simulink model "GreenCraneSimulator"  (R2021b)
settings: Solver=ode23  StartTime=0.0  StopTime=25  FixedStep=0.0001  RelTol=1e-3
undefined symbols (not defined in the file): Annulus_area, beta_F, Bore_area, cyl_c_end, cyl_c_visc, cyl_CH_stat, cyl_F_coul, cyl_FH_stat, cyl_gamma, cyl_k_end, DiscIntNeverNeededParam, dr_dcv, Eff_Bulk_On, eta_air, k_cv, k_DCV_PA, k_DCV_PB, k_DCV_T, k_ocv, K_oil, k_tanh, kappa_air, mu_ocv, OL_pa, OL_pb, p0_A, p0_A1, p0_B, p_cv_fo, p_cv_set, p_ocv_fo, p_ocv_set, p_pc_set, p_R, p_S, patm, Stroke, tau_ocv, tau_pc, tCycle, UL_at, UL_bt, V_CH_A, V_CH_A1, V_CH_B, v_cyl_0, wn_dcv, X, x_cyl_0, Y, Z
libraries: sm_lib x25, nesl_utility x4, simulink x1
(part 1 of 2)
settings Model: Creator=hagen  LastModifiedBy=danielh

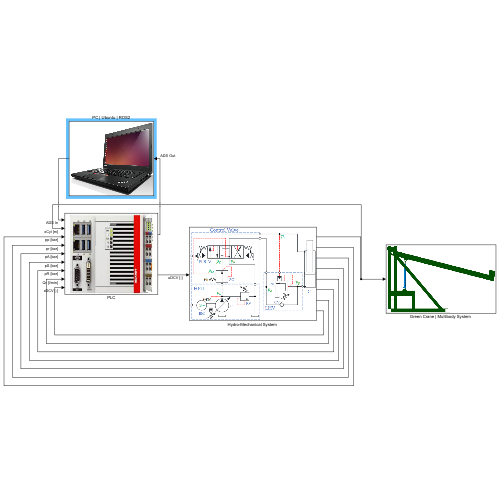
[thumbnail: Simulink's stored preview of the top-level diagram]
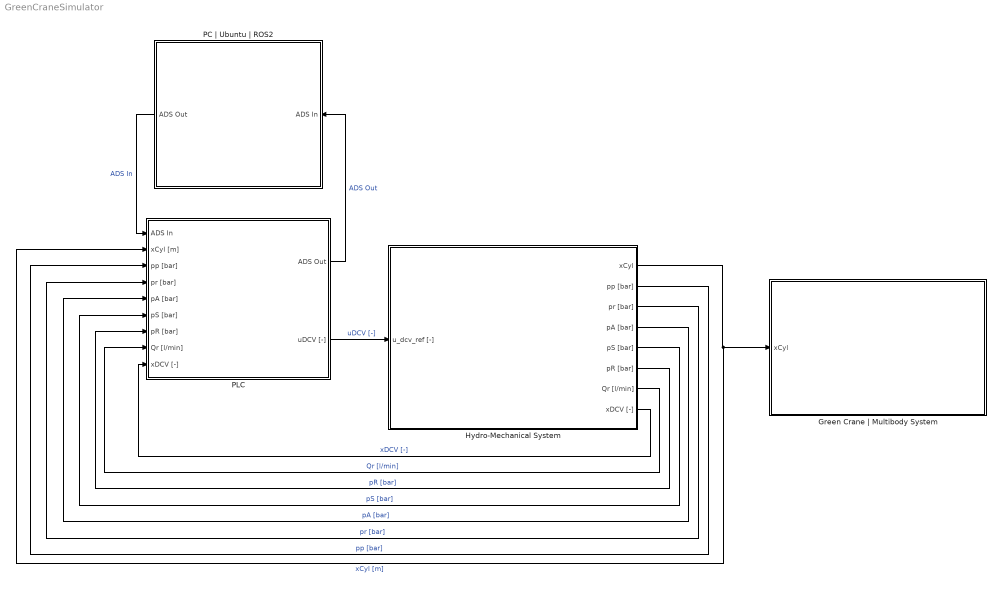
== system GreenCraneSimulator ==
  "Green Crane | Multibody System " : Subsystem
      mask Display: image('..\Simulink Model MAS418 LAB #11\Figures\GreenCrane.png'); % Use "Edit Image" on toolstrip to change.
  "Hydro-Mechanical System " : Subsystem
      mask Display: image('..\Simulink Model MAS418 LAB #11\Figures\HydroMechanicalSystem.png'); % Use "Edit Image" on toolstrip to change.
  PC | Ubuntu | ROS2 : Subsystem
      mask Display: image('..\Simulink Model MAS418 LAB #11\Figures\PC.png'); % Use "Edit Image" on toolstrip to change.
  PLC : Subsystem
      mask Display: image('..\Simulink Model MAS418 LAB #11\Figures\PLC.jpg'); % Use "Edit Image" on toolstrip to change.
  wires:
  PC | Ubuntu | ROS2/1(ADS Out) -> PLC/1(ADS In)  "ADS In"
  "Hydro-Mechanical System "/2(pp [bar]) -> PLC/3(pp [bar])  "pp [bar]"
  "Hydro-Mechanical System "/3(pr [bar]) -> PLC/4(pr [bar])  "pr [bar]"
  PLC/1(ADS Out) -> PC | Ubuntu | ROS2/1(ADS In)  "ADS Out"
  PLC/2(uDCV [-]) -> "Hydro-Mechanical System "/1(u_dcv_ref [-])  "uDCV [-]"
  "Hydro-Mechanical System "/4(pA [bar]) -> PLC/5(pA [bar])  "pA [bar]"
  "Hydro-Mechanical System "/8(xDCV [-]) -> PLC/9(xDCV [-])  "xDCV [-]"
  "Hydro-Mechanical System "/7(Qr [l/min]) -> PLC/8(Qr [l/min])  "Qr [l/min]"
  "Hydro-Mechanical System "/6(pR [bar]) -> PLC/7(pR [bar])  "pR [bar]"
  "Hydro-Mechanical System "/5(pS [bar]) -> PLC/6(pS [bar])  "pS [bar]"
  "Hydro-Mechanical System "/1(xCyl) -> PLC/2(xCyl [m]), "Green Crane | Multibody System "/1(xCyl)  "xCyl [m]"

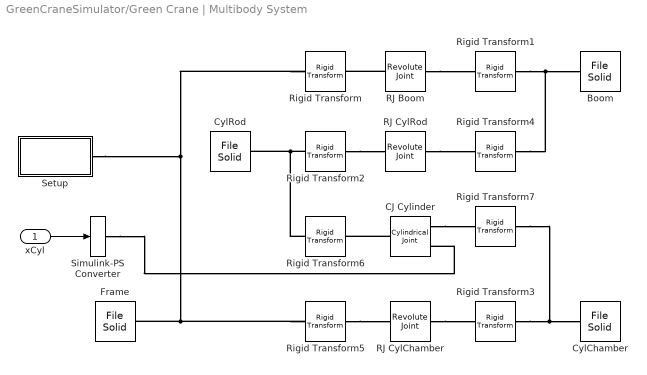
== system GreenCraneSimulator/Green Crane | Multibody System  ==
  xCyl : Inport
  Boom : sm_lib/Body Elements/File Solid  ExtGeomFileName=..\Simulink Model MAS418 LAB #7\CAD\Boom.STL  UnitType=Custom  ExtGeomFileUnits=mm  StepReaderType=HEX  ExportConvexHullGeometry=off  InertiaType=CalculateFromGeometry  Mass=1  MassUnits=kg  CenterOfMass=[0 0 0]  CenterOfMassUnits=m  MomentsOfInertia=[1 1 1]  MomentsOfInertiaUnits=kg*m^2  ProductsOfInertia=[0 0 0]  ProductsOfInertiaUnits=kg*m^2  BasedOnType=Density  Density=1000  DensityUnits=kg/m^3  DoExposeReferenceFrame=off  SerializedFrames=<Frames><Frame><Id>Frame1</Id><Value><Name>F1</Name><Origin><Source>CenterOfMassFrame</Source><FeatureName></FeatureName></Origin><PrimaryAxis><DefinedDirection>+Y</DefinedDirection><Source>ReferenceFrame</Source><SourceDirection>-Z</SourceDirection><FeatureName></FeatureName></PrimaryAxis><SecondaryAxis><DefinedDirection>+X</DefinedDirection><Source>ReferenceFrame</Source><SourceDirection>+X</SourceDirection><FeatureName></FeatureName></SecondaryAxis></Value></Frame></Frames>  GraphicType=FromGeometry  MarkerShape=Sphere  MarkerSize=10  GraphicVisPropType=SimpleVisualProperties  GraphicDiffuseColor=[0.0 0.4 0.0]  GraphicSpecularColor=[0.5 0.5 0.5 1.0]  GraphicAmbientColor=[0.15 0.15 0.15 1.0]  GraphicEmissiveColor=[0.0 0.0 0.0 1.0]  GraphicShininess=75  GraphicOpacity=1.0
  CJ Cylinder : sm_lib/Joints/Cylindrical Joint  JointMode=Normal  SenseConstraintForce=off  SenseConstraintForceX=off  SenseConstraintForceY=off  SenseConstraintForceZ=off  SenseConstraintTorque=off  SenseConstraintTorqueX=off  SenseConstraintTorqueY=off  SenseConstraintTorqueZ=off  SenseTotalForce=off  SenseTotalForceX=off  SenseTotalForceY=off  SenseTotalForceZ=off  SenseTotalTorque=off  SenseTotalTorqueX=off  SenseTotalTorqueY=off  SenseTotalTorqueZ=off  CompositeWrenchDir=FollowerOnBase  CompositeWrenchFrame=BaseFrame  PzEquilibriumPosition=0  PzEquilibriumPositionUnits=m  PzSpringStiffness=0  PzSpringStiffnessUnits=N/m  PzDampingCoefficient=0  PzDampingCoefficientUnits=N/(m/s)  PzTorqueActuationMode=ComputedTorque  PzMotionActuationMode=InputMotion  PzSensePosition=off  PzSenseVelocity=off  PzSenseAcceleration=off  PzSenseTorqueForce=off  PzSenseLowerLimitTorqueForce=off  PzSenseUpperLimitTorqueForce=off  PzLowerLimitSpecify=off  PzLowerLimitBound=-1  PzLowerLimitBoundUnits=m  PzLowerLimitStiffness=1e6  PzLowerLimitStiffnessUnits=N/m  PzLowerLimitDamping=1e3  PzLowerLimitDampingUnits=N/(m/s)  PzLowerLimitTransitionRegionWidth=1e-4  PzLowerLimitTransitionRegionWidthUnits=m  PzUpperLimitSpecify=off  PzUpperLimitBound=1  PzUpperLimitBoundUnits=m  PzUpperLimitStiffness=1e6  PzUpperLimitStiffnessUnits=N/m  PzUpperLimitDamping=1e3  PzUpperLimitDampingUnits=N/(m/s)  PzUpperLimitTransitionRegionWidth=1e-4  PzUpperLimitTransitionRegionWidthUnits=m  PzPositionTargetSpecify=on  PzPositionTargetPriority=High  PzPositionTargetValue=x_cyl_0  PzPositionTargetValueUnits=m  PzVelocityTargetSpecify=off  PzVelocityTargetPriority=High  PzVelocityTargetValue=0  PzVelocityTargetValueUnits=m/s  RzEquilibriumPosition=0  RzEquilibriumPositionUnits=deg  RzSpringStiffness=0  RzSpringStiffnessUnits=N*m/deg  RzDampingCoefficient=0  RzDampingCoefficientUnits=N*m/(deg/s)  RzTorqueActuationMode=NoTorque  RzMotionActuationMode=ComputedMotion  RzSensePosition=off  RzSenseVelocity=off  RzSenseAcceleration=off  RzSenseTorqueForce=off  RzSenseLowerLimitTorqueForce=off  RzSenseUpperLimitTorqueForce=off  RzLowerLimitSpecify=off  RzLowerLimitBound=-90  RzLowerLimitBoundUnits=deg  RzLowerLimitStiffness=1e4  RzLowerLimitStiffnessUnits=N*m/deg  RzLowerLimitDamping=10  RzLowerLimitDampingUnits=N*m/(deg/s)  RzLowerLimitTransitionRegionWidth=0.1  RzLowerLimitTransitionRegionWidthUnits=deg  RzUpperLimitSpecify=off  RzUpperLimitBound=90  RzUpperLimitBoundUnits=deg  RzUpperLimitStiffness=1e4  RzUpperLimitStiffnessUnits=N*m/deg  RzUpperLimitDamping=10  RzUpperLimitDampingUnits=N*m/(deg/s)  RzUpperLimitTransitionRegionWidth=0.1  RzUpperLimitTransitionRegionWidthUnits=deg  RzPositionTargetSpecify=off  RzPositionTargetPriority=High  RzPositionTargetValue=0  RzPositionTargetValueUnits=deg  RzVelocityTargetSpecify=off  RzVelocityTargetPriority=High  RzVelocityTargetValue=0  RzVelocityTargetValueUnits=deg/s
  CylChamber : sm_lib/Body Elements/File Solid  ExtGeomFileName=..\Simulink Model MAS418 LAB #7\CAD\cyl_chamber.STL  UnitType=Custom  ExtGeomFileUnits=mm  StepReaderType=HEX  ExportConvexHullGeometry=off  InertiaType=CalculateFromGeometry  Mass=1  MassUnits=kg  CenterOfMass=[0 0 0]  CenterOfMassUnits=m  MomentsOfInertia=[1 1 1]  MomentsOfInertiaUnits=kg*m^2  ProductsOfInertia=[0 0 0]  ProductsOfInertiaUnits=kg*m^2  BasedOnType=Density  Density=1000  DensityUnits=kg/m^3  DoExposeReferenceFrame=off  SerializedFrames=<Frames><Frame><Id>Frame1</Id><Value><Name>F1</Name><Origin><Source>CenterOfMassFrame</Source><FeatureName></FeatureName></Origin><PrimaryAxis><DefinedDirection>+Y</DefinedDirection><Source>ReferenceFrame</Source><SourceDirection>-Z</SourceDirection><FeatureName></FeatureName></PrimaryAxis><SecondaryAxis><DefinedDirection>+X</DefinedDirection><Source>ReferenceFrame</Source><SourceDirection>+X</SourceDirection><FeatureName></FeatureName></SecondaryAxis></Value></Frame></Frames>  GraphicType=FromGeometry  MarkerShape=Sphere  MarkerSize=10  GraphicVisPropType=SimpleVisualProperties  GraphicDiffuseColor=[0.0 0.6 1.0]  GraphicSpecularColor=[0.5 0.5 0.5 1.0]  GraphicAmbientColor=[0.15 0.15 0.15 1.0]  GraphicEmissiveColor=[0.0 0.0 0.0 1.0]  GraphicShininess=75  GraphicOpacity=1.0
  CylRod : sm_lib/Body Elements/File Solid  ExtGeomFileName=..\Simulink Model MAS418 LAB #7\CAD\cyl_rod.STL  UnitType=Custom  ExtGeomFileUnits=mm  StepReaderType=HEX  ExportConvexHullGeometry=off  InertiaType=CalculateFromGeometry  Mass=1  MassUnits=kg  CenterOfMass=[0 0 0]  CenterOfMassUnits=m  MomentsOfInertia=[1 1 1]  MomentsOfInertiaUnits=kg*m^2  ProductsOfInertia=[0 0 0]  ProductsOfInertiaUnits=kg*m^2  BasedOnType=Density  Density=1000  DensityUnits=kg/m^3  DoExposeReferenceFrame=off  SerializedFrames=<Frames><Frame><Id>Frame1</Id><Value><Name>F1</Name><Origin><Source>CenterOfMassFrame</Source><FeatureName></FeatureName></Origin><PrimaryAxis><DefinedDirection>+Y</DefinedDirection><Source>ReferenceFrame</Source><SourceDirection>-Z</SourceDirection><FeatureName></FeatureName></PrimaryAxis><SecondaryAxis><DefinedDirection>+X</DefinedDirection><Source>ReferenceFrame</Source><SourceDirection>+X</SourceDirection><FeatureName></FeatureName></SecondaryAxis></Value></Frame></Frames>  GraphicType=FromGeometry  MarkerShape=Sphere  MarkerSize=10  GraphicVisPropType=SimpleVisualProperties  GraphicDiffuseColor=[0.8 0.8 0.8]  GraphicSpecularColor=[0.5 0.5 0.5 1.0]  GraphicAmbientColor=[0.15 0.15 0.15 1.0]  GraphicEmissiveColor=[0.0 0.0 0.0 1.0]  GraphicShininess=75  GraphicOpacity=1.0
  Frame : sm_lib/Body Elements/File Solid  ExtGeomFileName=..\Simulink Model MAS418 LAB #7\CAD\Frame.STL  UnitType=Custom  ExtGeomFileUnits=mm  StepReaderType=HEX  ExportConvexHullGeometry=off  InertiaType=CalculateFromGeometry  Mass=1  MassUnits=kg  CenterOfMass=[0 0 0]  CenterOfMassUnits=m  MomentsOfInertia=[1 1 1]  MomentsOfInertiaUnits=kg*m^2  ProductsOfInertia=[0 0 0]  ProductsOfInertiaUnits=kg*m^2  BasedOnType=Density  Density=1000  DensityUnits=kg/m^3  DoExposeReferenceFrame=off  SerializedFrames=<Frames><Frame><Id>Frame1</Id><Value><Name>F1</Name><Origin><Source>CenterOfMassFrame</Source><FeatureName></FeatureName></Origin><PrimaryAxis><DefinedDirection>-Y</DefinedDirection><Source>ReferenceFrame</Source><SourceDirection>+Z</SourceDirection><FeatureName></FeatureName></PrimaryAxis><SecondaryAxis><DefinedDirection>+X</DefinedDirection><Source>ReferenceFrame</Source><SourceDirection>+X</SourceDirection><FeatureName></FeatureName></SecondaryAxis></Value></Frame></Frames>  GraphicType=FromGeometry  MarkerShape=Sphere  MarkerSize=10  GraphicVisPropType=SimpleVisualProperties  GraphicDiffuseColor=[0.0 0.4 0.0]  GraphicSpecularColor=[0.5 0.5 0.5 1.0]  GraphicAmbientColor=[0.15 0.15 0.15 1.0]  GraphicEmissiveColor=[0.0 0.0 0.0 1.0]  GraphicShininess=75  GraphicOpacity=1.0
  RJ Boom : sm_lib/Joints/Revolute Joint  JointMode=Normal  SenseConstraintForce=off  SenseConstraintForceX=off  SenseConstraintForceY=off  SenseConstraintForceZ=off  SenseConstraintTorque=off  SenseConstraintTorqueX=off  SenseConstraintTorqueY=off  SenseConstraintTorqueZ=off  SenseTotalForce=off  SenseTotalForceX=off  SenseTotalForceY=off  SenseTotalForceZ=off  SenseTotalTorque=off  SenseTotalTorqueX=off  SenseTotalTorqueY=off  SenseTotalTorqueZ=off  CompositeWrenchDir=FollowerOnBase  CompositeWrenchFrame=BaseFrame  EquilibriumPosition=0  EquilibriumPositionUnits=deg  SpringStiffness=0  SpringStiffnessUnits=N*m/deg  DampingCoefficient=0  DampingCoefficientUnits=N*m/(deg/s)  TorqueActuationMode=NoTorque  MotionActuationMode=ComputedMotion  SensePosition=off  SenseVelocity=off  SenseAcceleration=off  SenseTorqueForce=off  SenseLowerLimitTorqueForce=off  SenseUpperLimitTorqueForce=off  LowerLimitSpecify=off  LowerLimitBound=-90  LowerLimitBoundUnits=deg  LowerLimitStiffness=1e4  LowerLimitStiffnessUnits=N*m/deg  LowerLimitDamping=10  LowerLimitDampingUnits=N*m/(deg/s)  LowerLimitTransitionRegionWidth=0.1  LowerLimitTransitionRegionWidthUnits=deg  UpperLimitSpecify=off  UpperLimitBound=90  UpperLimitBoundUnits=deg  UpperLimitStiffness=1e4  UpperLimitStiffnessUnits=N*m/deg  UpperLimitDamping=10  UpperLimitDampingUnits=N*m/(deg/s)  UpperLimitTransitionRegionWidth=0.1  UpperLimitTransitionRegionWidthUnits=deg  PositionTargetSpecify=off  PositionTargetPriority=High  PositionTargetValue=0  PositionTargetValueUnits=deg  VelocityTargetSpecify=off  VelocityTargetPriority=High  VelocityTargetValue=0  VelocityTargetValueUnits=deg/s
  RJ CylChamber : sm_lib/Joints/Revolute Joint  JointMode=Normal  SenseConstraintForce=off  SenseConstraintForceX=off  SenseConstraintForceY=off  SenseConstraintForceZ=off  SenseConstraintTorque=off  SenseConstraintTorqueX=off  SenseConstraintTorqueY=off  SenseConstraintTorqueZ=off  SenseTotalForce=off  SenseTotalForceX=off  SenseTotalForceY=off  SenseTotalForceZ=off  SenseTotalTorque=off  SenseTotalTorqueX=off  SenseTotalTorqueY=off  SenseTotalTorqueZ=off  CompositeWrenchDir=FollowerOnBase  CompositeWrenchFrame=BaseFrame  EquilibriumPosition=0  EquilibriumPositionUnits=deg  SpringStiffness=0  SpringStiffnessUnits=N*m/deg  DampingCoefficient=0  DampingCoefficientUnits=N*m/(deg/s)  TorqueActuationMode=NoTorque  MotionActuationMode=ComputedMotion  SensePosition=off  SenseVelocity=off  SenseAcceleration=off  SenseTorqueForce=off  SenseLowerLimitTorqueForce=off  SenseUpperLimitTorqueForce=off  LowerLimitSpecify=off  LowerLimitBound=-90  LowerLimitBoundUnits=deg  LowerLimitStiffness=1e4  LowerLimitStiffnessUnits=N*m/deg  LowerLimitDamping=10  LowerLimitDampingUnits=N*m/(deg/s)  LowerLimitTransitionRegionWidth=0.1  LowerLimitTransitionRegionWidthUnits=deg  UpperLimitSpecify=off  UpperLimitBound=90  UpperLimitBoundUnits=deg  UpperLimitStiffness=1e4  UpperLimitStiffnessUnits=N*m/deg  UpperLimitDamping=10  UpperLimitDampingUnits=N*m/(deg/s)  UpperLimitTransitionRegionWidth=0.1  UpperLimitTransitionRegionWidthUnits=deg  PositionTargetSpecify=off  PositionTargetPriority=High  PositionTargetValue=0  PositionTargetValueUnits=deg  VelocityTargetSpecify=off  VelocityTargetPriority=High  VelocityTargetValue=0  VelocityTargetValueUnits=deg/s
  RJ CylRod : sm_lib/Joints/Revolute Joint  JointMode=Normal  SenseConstraintForce=off  SenseConstraintForceX=off  SenseConstraintForceY=off  SenseConstraintForceZ=off  SenseConstraintTorque=off  SenseConstraintTorqueX=off  SenseConstraintTorqueY=off  SenseConstraintTorqueZ=off  SenseTotalForce=off  SenseTotalForceX=off  SenseTotalForceY=off  SenseTotalForceZ=off  SenseTotalTorque=off  SenseTotalTorqueX=off  SenseTotalTorqueY=off  SenseTotalTorqueZ=off  CompositeWrenchDir=FollowerOnBase  CompositeWrenchFrame=BaseFrame  EquilibriumPosition=0  EquilibriumPositionUnits=deg  SpringStiffness=0  SpringStiffnessUnits=N*m/deg  DampingCoefficient=0  DampingCoefficientUnits=N*m/(deg/s)  TorqueActuationMode=NoTorque  MotionActuationMode=ComputedMotion  SensePosition=off  SenseVelocity=off  SenseAcceleration=off  SenseTorqueForce=off  SenseLowerLimitTorqueForce=off  SenseUpperLimitTorqueForce=off  LowerLimitSpecify=off  LowerLimitBound=-90  LowerLimitBoundUnits=deg  LowerLimitStiffness=1e4  LowerLimitStiffnessUnits=N*m/deg  LowerLimitDamping=10  LowerLimitDampingUnits=N*m/(deg/s)  LowerLimitTransitionRegionWidth=0.1  LowerLimitTransitionRegionWidthUnits=deg  UpperLimitSpecify=off  UpperLimitBound=90  UpperLimitBoundUnits=deg  UpperLimitStiffness=1e4  UpperLimitStiffnessUnits=N*m/deg  UpperLimitDamping=10  UpperLimitDampingUnits=N*m/(deg/s)  UpperLimitTransitionRegionWidth=0.1  UpperLimitTransitionRegionWidthUnits=deg  PositionTargetSpecify=off  PositionTargetPriority=High  PositionTargetValue=0  PositionTargetValueUnits=deg  VelocityTargetSpecify=off  VelocityTargetPriority=High  VelocityTargetValue=0  VelocityTargetValueUnits=deg/s
  Rigid Transform : sm_lib/Frames and Transforms/Rigid Transform  TranslationMethod=Cartesian  TranslationStandardOffset=0  TranslationLengthUnit=mm  TranslationStandardAxis=+Z  TranslationCartesianOffset=[-568.76 0 1179.93]  TranslationROffset=0  TranslationROffsetUnits=m  TranslationZOffset=0  TranslationZOffsetUnits=m  TranslationThetaOffset=0  TranslationThetaOffsetUnits=deg  RotationMethod=StandardAxis  RotationAngleUnits=deg  RotationStandardAxis=+X  RotationAngle=90  RotationArbitraryAxis=[0 0 1]  FollAlignAxisA=+X  BaseAlignAxisA=+Y  FollAlignAxisB=+Y  BaseAlignAxisB=+Z  RotationSequenceAxes=FollowerAxes  RotationSequence=XYX  RotationSequenceAngles=[0 0 0]  RotationSequenceAnglesUnits=deg  RotationMatrix=[1 0 0; 0 1 0; 0 0 1]
  Rigid Transform1 : sm_lib/Frames and Transforms/Rigid Transform  TranslationMethod=Cartesian  TranslationStandardOffset=0  TranslationLengthUnit=mm  TranslationStandardAxis=+Z  TranslationCartesianOffset=[-3108.36 0 -63.43]  TranslationROffset=0  TranslationROffsetUnits=m  TranslationZOffset=0  TranslationZOffsetUnits=m  TranslationThetaOffset=0  TranslationThetaOffsetUnits=deg  RotationMethod=StandardAxis  RotationAngleUnits=deg  RotationStandardAxis=+X  RotationAngle=90  RotationArbitraryAxis=[0 0 1]  FollAlignAxisA=+X  BaseAlignAxisA=+Y  FollAlignAxisB=+Y  BaseAlignAxisB=+Z  RotationSequenceAxes=FollowerAxes  RotationSequence=XYX  RotationSequenceAngles=[0 0 0]  RotationSequenceAnglesUnits=deg  RotationMatrix=[1 0 0; 0 1 0; 0 0 1]
  Rigid Transform2 : sm_lib/Frames and Transforms/Rigid Transform  TranslationMethod=Cartesian  TranslationStandardOffset=0  TranslationLengthUnit=mm  TranslationStandardAxis=+Z  TranslationCartesianOffset=[0 0 292.43]  TranslationROffset=0  TranslationROffsetUnits=m  TranslationZOffset=0  TranslationZOffsetUnits=m  TranslationThetaOffset=0  TranslationThetaOffsetUnits=deg  RotationMethod=StandardAxis  RotationAngleUnits=deg  RotationStandardAxis=+X  RotationAngle=90  RotationArbitraryAxis=[0 0 1]  FollAlignAxisA=+X  BaseAlignAxisA=+Y  FollAlignAxisB=+Y  BaseAlignAxisB=+Z  RotationSequenceAxes=FollowerAxes  RotationSequence=XYX  RotationSequenceAngles=[0 0 0]  RotationSequenceAnglesUnits=deg  RotationMatrix=[1 0 0; 0 1 0; 0 0 1]
  Rigid Transform3 : sm_lib/Frames and Transforms/Rigid Transform  TranslationMethod=Cartesian  TranslationStandardOffset=0  TranslationLengthUnit=mm  TranslationStandardAxis=+Z  TranslationCartesianOffset=[0 0 -260.99]  TranslationROffset=0  TranslationROffsetUnits=m  TranslationZOffset=0  TranslationZOffsetUnits=m  TranslationThetaOffset=0  TranslationThetaOffsetUnits=deg  RotationMethod=StandardAxis  RotationAngleUnits=deg  RotationStandardAxis=+X  RotationAngle=90  RotationArbitraryAxis=[0 0 1]  FollAlignAxisA=+X  BaseAlignAxisA=+Y  FollAlignAxisB=+Y  BaseAlignAxisB=+Z  RotationSequenceAxes=FollowerAxes  RotationSequence=XYX  RotationSequenceAngles=[0 0 0]  RotationSequenceAnglesUnits=deg  RotationMatrix=[1 0 0; 0 1 0; 0 0 1]
  Rigid Transform4 : sm_lib/Frames and Transforms/Rigid Transform  TranslationMethod=Cartesian  TranslationStandardOffset=0  TranslationLengthUnit=mm  TranslationStandardAxis=+Z  TranslationCartesianOffset=[-2613.52 0 -196.43]  TranslationROffset=0  TranslationROffsetUnits=m  TranslationZOffset=0  TranslationZOffsetUnits=m  TranslationThetaOffset=0  TranslationThetaOffsetUnits=deg  RotationMethod=StandardAxis  RotationAngleUnits=deg  RotationStandardAxis=+X  RotationAngle=90  RotationArbitraryAxis=[0 0 1]  FollAlignAxisA=+X  BaseAlignAxisA=+Y  FollAlignAxisB=+Y  BaseAlignAxisB=+Z  RotationSequenceAxes=FollowerAxes  RotationSequence=XYX  RotationSequenceAngles=[0 0 0]  RotationSequenceAnglesUnits=deg  RotationMatrix=[1 0 0; 0 1 0; 0 0 1]
  Rigid Transform5 : sm_lib/Frames and Transforms/Rigid Transform  TranslationMethod=Cartesian  TranslationStandardOffset=0  TranslationLengthUnit=mm  TranslationStandardAxis=+Z  TranslationCartesianOffset=[-141.76 0 122.93]  TranslationROffset=0  TranslationROffsetUnits=m  TranslationZOffset=0  TranslationZOffsetUnits=m  TranslationThetaOffset=0  TranslationThetaOffsetUnits=deg  RotationMethod=StandardAxis  RotationAngleUnits=deg  RotationStandardAxis=+X  RotationAngle=90  RotationArbitraryAxis=[0 0 1]  FollAlignAxisA=+X  BaseAlignAxisA=+Y  FollAlignAxisB=+Y  BaseAlignAxisB=+Z  RotationSequenceAxes=FollowerAxes  RotationSequence=XYX  RotationSequenceAngles=[0 0 0]  RotationSequenceAnglesUnits=deg  RotationMatrix=[1 0 0; 0 1 0; 0 0 1]
  Rigid Transform6 : sm_lib/Frames and Transforms/Rigid Transform  TranslationMethod=Cartesian  TranslationStandardOffset=0  TranslationLengthUnit=mm  TranslationStandardAxis=+Z  TranslationCartesianOffset=[0 0 -307.79]  TranslationROffset=0  TranslationROffsetUnits=m  TranslationZOffset=0  TranslationZOffsetUnits=m  TranslationThetaOffset=0  TranslationThetaOffsetUnits=deg  RotationMethod=None  RotationAngleUnits=deg  RotationStandardAxis=-X  RotationAngle=90  RotationArbitraryAxis=[0 0 1]  FollAlignAxisA=+X  BaseAlignAxisA=+Y  FollAlignAxisB=+Y  BaseAlignAxisB=+Z  RotationSequenceAxes=FollowerAxes  RotationSequence=XYX  RotationSequenceAngles=[0 0 0]  RotationSequenceAnglesUnits=deg  RotationMatrix=[1 0 0; 0 1 0; 0 0 1]
  Rigid Transform7 : sm_lib/Frames and Transforms/Rigid Transform  TranslationMethod=Cartesian  TranslationStandardOffset=0  TranslationLengthUnit=mm  TranslationStandardAxis=+Z  TranslationCartesianOffset=[0 0 -88.99]  TranslationROffset=0  TranslationROffsetUnits=m  TranslationZOffset=0  TranslationZOffsetUnits=m  TranslationThetaOffset=0  TranslationThetaOffsetUnits=deg  RotationMethod=None  RotationAngleUnits=deg  RotationStandardAxis=-X  RotationAngle=90  RotationArbitraryAxis=[0 0 1]  FollAlignAxisA=+X  BaseAlignAxisA=+Y  FollAlignAxisB=+Y  BaseAlignAxisB=+Z  RotationSequenceAxes=FollowerAxes  RotationSequence=XYX  RotationSequenceAngles=[0 0 0]  RotationSequenceAnglesUnits=deg  RotationMatrix=[1 0 0; 0 1 0; 0 0 1]
  Setup : Subsystem
  Simulink-PS Converter : nesl_utility/Simulink-PS Converter  PhysicalDomain=network_engine_domain  SubClassName=ps_input  LeftPortType=input  RightPortType=output  PseudoPeriodic=off  Frequencies=[]  NoiseDistribution=none  NoiseParameters=[]  Unit=1  AffineConversion=off  FilteringAndDerivatives=filter  SimscapeFilterOrder=2  InputFilterTimeConstant=0.001  UdotUserProvided=0
      settings: SourceProductBaseCode=PW,SS
  wires:
  xCyl/1 -> Simulink-PS Converter/1
  connections:
  Rigid Transform/LConn1 -- Rigid Transform5/LConn1 -- Frame/LConn1 -- Setup/RConn1
  CJ Cylinder/LConn1 -- Rigid Transform7/RConn1
  Rigid Transform2/LConn1 -- Rigid Transform6/LConn1 -- CylRod/LConn1
  Rigid Transform1/LConn1 -- Rigid Transform4/LConn1 -- Boom/LConn1
  Rigid Transform3/LConn1 -- Rigid Transform7/LConn1 -- CylChamber/LConn1
  RJ CylChamber/RConn1 -- Rigid Transform3/RConn1
  RJ Boom/LConn1 -- Rigid Transform/RConn1
  CJ Cylinder/RConn1 -- Rigid Transform6/RConn1
  RJ Boom/RConn1 -- Rigid Transform1/RConn1
  Simulink-PS Converter/RConn1 -- CJ Cylinder/LConn2
  Rigid Transform5/RConn1 -- RJ CylChamber/LConn1
  RJ CylRod/LConn1 -- Rigid Transform4/RConn1
  Rigid Transform2/RConn1 -- RJ CylRod/RConn1

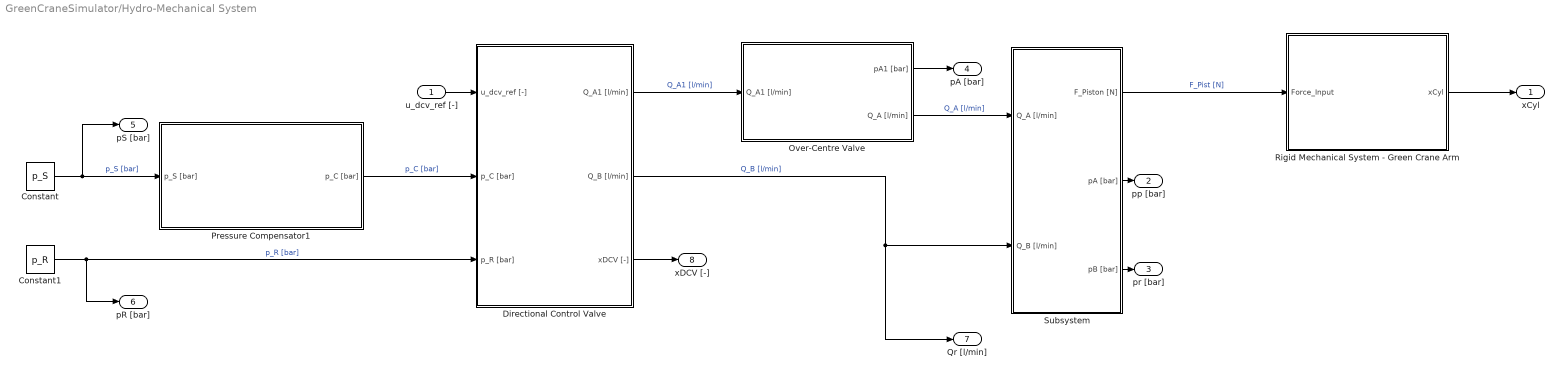
== system GreenCraneSimulator/Hydro-Mechanical System  ==
  u_dcv_ref [-] : Inport
  Constant : Constant  Value=p_S
  Constant1 : Constant  Value=p_R
  Directional Control Valve : Subsystem
      mask Display: disp('{\bf\fontsize{22}Directional\newline Control Valve}', 'texmode','on');
  Over-Centre Valve : Subsystem
      mask Display: disp('{\bf\fontsize{22}Load-Holding\newline Valve}', 'texmode','on');
  Pressure Compensator1 : Subsystem
      mask Display: disp('{\bf\fontsize{22}Pressure\newline Compensator}', 'texmode','on');
  Rigid Mechanical System - Green Crane Arm : Subsystem  VariantControl=Rigid_model
  Subsystem : Subsystem
      mask Display: disp('{\bf\fontsize{22} Hydraulic \newline Cylinder}', 'texmode','on');
  xCyl : Outport
  pp [bar] : Outport  Port=2  VectorParamsAs1DForOutWhenUnconnected=off
  pr [bar] : Outport  Port=3  VectorParamsAs1DForOutWhenUnconnected=off
  pA [bar] : Outport  Port=4  VectorParamsAs1DForOutWhenUnconnected=off
  pS [bar] : Outport  Port=5  VectorParamsAs1DForOutWhenUnconnected=off
  pR [bar] : Outport  Port=6  VectorParamsAs1DForOutWhenUnconnected=off
  Qr [l/min] : Outport  Port=7  VectorParamsAs1DForOutWhenUnconnected=off
  xDCV [-] : Outport  Port=8  VectorParamsAs1DForOutWhenUnconnected=off
  wires:
  Subsystem/1(F_Piston [N]) -> Rigid Mechanical System - Green Crane Arm/1(Force_Input)  "F_Pist [N]"
  Constant/1 -> pS [bar]/1, Pressure Compensator1/1(p_S [bar])  "p_S [bar]"
  Pressure Compensator1/1(p_C [bar]) -> Directional Control Valve/2(p_C [bar])  "p_C [bar]"
  Directional Control Valve/2(Q_B [l/min]) -> Qr [l/min]/1, Subsystem/2(Q_B [l/min])  "Q_B [l/min]"
  u_dcv_ref [-]/1 -> Directional Control Valve/1(u_dcv_ref [-])
  Over-Centre Valve/2(Q_A [l/min]) -> Subsystem/1(Q_A [l/min])  "Q_A [l/min]"
  Constant1/1 -> pR [bar]/1, Directional Control Valve/3(p_R [bar])  "p_R [bar]"
  Directional Control Valve/1(Q_A1 [l/min]) -> Over-Centre Valve/1(Q_A1 [l/min])  "Q_A1 [l/min]"
  Rigid Mechanical System - Green Crane Arm/1(xCyl) -> xCyl/1
  Subsystem/2(pA [bar]) -> pp [bar]/1
  Subsystem/3(pB [bar]) -> pr [bar]/1
  Over-Centre Valve/1(pA1 [bar]) -> pA [bar]/1
  Directional Control Valve/3(xDCV [-]) -> xDCV [-]/1

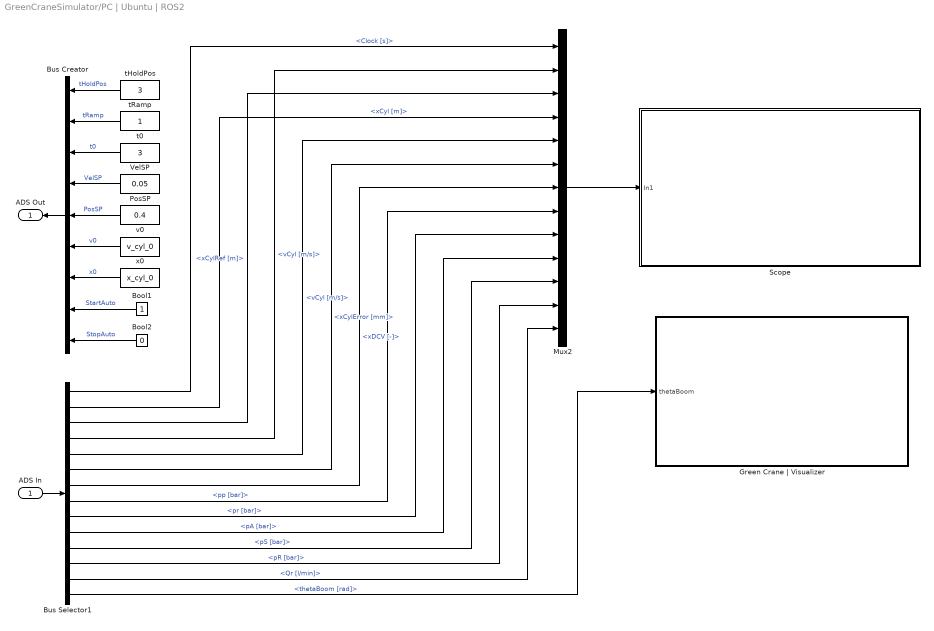
== system GreenCraneSimulator/PC | Ubuntu | ROS2 ==
  ADS In : Inport
  Bool1 : Constant  OutDataTypeStr=boolean
  Bool2 : Constant  Value=0  OutDataTypeStr=boolean
  Bus Creator : BusCreator  Inputs=9
  Bus Selector1 : BusSelector  OutputSignals=Clock [s],xCyl [m],xCylRef [m],vCyl [m/s],vCyl [m/s],xCylError [mm],xDCV [-],pp [bar],pr [bar],pA [bar],pS [bar],pR [bar],Qr [l/min],thetaBoom [rad]
  "Green Crane | Visualizer " : Subsystem
      mask Display: image('..\Simulink Model MAS418 LAB #11\Figures\GreenCraneSimple.png'); % Use "Edit Image" on toolstrip to change.
  Mux2 : Mux  Inputs=13
  PosSP : Constant  Value=0.4  OutDataTypeStr=double
  Scope : Subsystem
      mask Display: image('..\Simulink Model MAS418 LAB #11\Figures\Scope.png'); % Use "Edit Image" on toolstrip to change.
  VelSP : Constant  Value=0.05  OutDataTypeStr=double
  t0 : Constant  Value=3  OutDataTypeStr=double
  tHoldPos : Constant  Value=3  OutDataTypeStr=double
  tRamp : Constant  OutDataTypeStr=double
  v0 : Constant  Value=v_cyl_0  OutDataTypeStr=double
  x0 : Constant  Value=x_cyl_0  OutDataTypeStr=double
  ADS Out : Outport
  wires:
  Bus Selector1/1 -> Mux2/1  "<Clock [s]>"
  Bus Selector1/2 -> Mux2/4  "<xCyl [m]>"
  Bus Selector1/4 -> Mux2/2  "<vCyl [m/s]>"
  Bus Creator/1 -> ADS Out/1
  ADS In/1 -> Bus Selector1/1
  Bus Selector1/8 -> Mux2/8  "<pp [bar]>"
  Bus Selector1/9 -> Mux2/9  "<pr [bar]>"
  Bus Selector1/6 -> Mux2/6  "<xCylError [mm]>"
  Mux2/1 -> Scope/1(In1)
  Bus Selector1/10 -> Mux2/10  "<pA [bar]>"
  Bus Selector1/11 -> Mux2/11  "<pS [bar]>"
  Bus Selector1/12 -> Mux2/12  "<pR [bar]>"
  Bus Selector1/13 -> Mux2/13  "<Qr [l/min]>"
  Bus Selector1/7 -> Mux2/7  "<xDCV [-]>"
  Bus Selector1/14 -> "Green Crane | Visualizer "/1(thetaBoom)  "<thetaBoom [rad]>"
  tHoldPos/1 -> Bus Creator/1  "tHoldPos"
  tRamp/1 -> Bus Creator/2  "tRamp"
  t0/1 -> Bus Creator/3  "t0"
  VelSP/1 -> Bus Creator/4  "VelSP"
  PosSP/1 -> Bus Creator/5  "PosSP"
  v0/1 -> Bus Creator/6  "v0"
  x0/1 -> Bus Creator/7  "x0"
  Bus Selector1/3 -> Mux2/3  "<xCylRef [m]>"
  Bus Selector1/5 -> Mux2/5  "<vCyl [m/s]>"
  Bool1/1 -> Bus Creator/8  "StartAuto"
  Bool2/1 -> Bus Creator/9  "StopAuto"

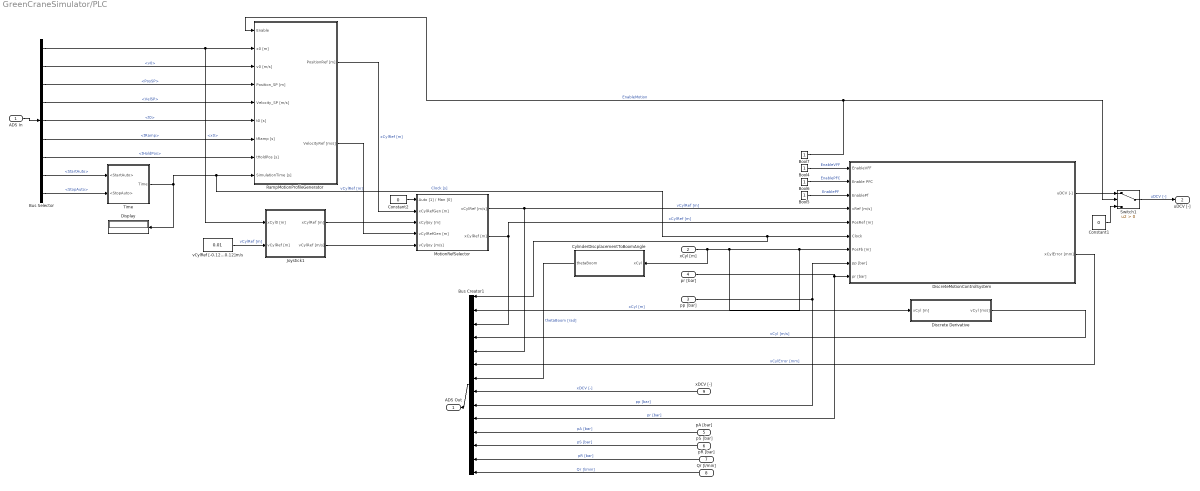
== system GreenCraneSimulator/PLC ==
  ADS In : Inport
  xCyl [m] : Inport  Port=2
  pp [bar] : Inport  Port=3
  pr [bar] : Inport  Port=4
  pA [bar] : Inport  Port=5
  pS [bar] : Inport  Port=6
  pR [bar] : Inport  Port=7
  Qr [l/min] : Inport  Port=8
  xDCV [-] : Inport  Port=9
  Bool{4..7} (4 alike) : Constant  OutDataTypeStr=boolean
  Bus Creator1 : BusCreator  Inputs=14
  Bus Selector : BusSelector  OutputSignals=x0,v0,PosSP,VelSP,t0,tRamp,tHoldPos,StartAuto,StopAuto
  Constant1 : Constant  Value=0
  Constant2 : Constant  Value=0  OutDataTypeStr=boolean
  CylinderDiscplacementToBoomAngle : MATLAB Function  TreatAsAtomicUnit=on
  Discrete Derivative : Subsystem
  DiscreteMotionControlSystem : Subsystem
      mask Display: image('..\Simulink Model MAS418 LAB #11\Figures\MotionControlSystem.png'); % Use "Edit Image" on toolstrip to change.
  Display : Display
  Joystick1 : Subsystem
  MotionRefSelector : Subsystem
  RampMotionProfileGenerator : Subsystem  TreatAsAtomicUnit=on  VariantControl=Ramp_Profile
  Switch1 : Switch  Criteria=u2 > Threshold
  Time : Subsystem
  vCylRef [-0.12...0.12]m/s : Constant  Value=0.01  OutDataTypeStr=double
  ADS Out : Outport
  uDCV [-] : Outport  Port=2
  wires:
  Switch1/1 -> uDCV [-]/1  "uDCV [-]"
  xCyl [m]/1 -> CylinderDiscplacementToBoomAngle/1(xCyl), Discrete Derivative/1(xCyl [m]), Bus Creator1/2, DiscreteMotionControlSystem/7(PosFb [m])  "xCyl [m]"
  pr [bar]/1 -> Bus Creator1/10, DiscreteMotionControlSystem/9(pr [bar])  "pr [bar]"
  Time/1(Time) -> Display/1, Bus Creator1/1, DiscreteMotionControlSystem/6(Clock), RampMotionProfileGenerator/9(SimulationTime [s])  "Clock [s]"
  pp [bar]/1 -> Bus Creator1/9, DiscreteMotionControlSystem/8(pp [bar])  "pp [bar]"
  Bus Creator1/1 -> ADS Out/1
  ADS In/1 -> Bus Selector/1
  Constant1/1 -> Switch1/3
  DiscreteMotionControlSystem/1(uDCV [-]) -> Switch1/1
  DiscreteMotionControlSystem/2(xCylError [mm]) -> Bus Creator1/6  "xCylError [mm]"
  Discrete Derivative/1(vCyl [m/s]) -> Bus Creator1/4  "vCyl [m/s]"
  xDCV [-]/1 -> Bus Creator1/8  "xDCV [-]"
  pA [bar]/1 -> Bus Creator1/11  "pA [bar]"
  pS [bar]/1 -> Bus Creator1/12  "pS [bar]"
  pR [bar]/1 -> Bus Creator1/13  "pR [bar]"
  Qr [l/min]/1 -> Bus Creator1/14  "Qr [l/min]"
  CylinderDiscplacementToBoomAngle/1(thetaBoom) -> Bus Creator1/7  "thetaBoom [rad]"
  vCylRef [-0.12...0.12]m/s/1 -> Joystick1/2(vCylRef [m])  "vCylRef [m]"
  Bus Selector/1 -> RampMotionProfileGenerator/2(x0 [m]), Joystick1/1(xCyl0 [m])  "<x0>"
  Joystick1/2(vCylRef [m/s]) -> MotionRefSelector/5(vCylJoy [m/s])
  Constant2/1 -> MotionRefSelector/1(Auto [1] / Man [0])
  Joystick1/1(xCylRef [m]) -> MotionRefSelector/3(xCylJoy [m])
  RampMotionProfileGenerator/1("PositionRef [m] ") -> MotionRefSelector/2(xCylRefGen [m])  "xCylRef [m]"
  Bus Selector/5 -> RampMotionProfileGenerator/6(t0 [s])  "<t0>"
  MotionRefSelector/1(vCylRef [m/s]) -> Bus Creator1/5, DiscreteMotionControlSystem/4(vRef [m/s])  "vCylRef [m]"
  Bus Selector/2 -> RampMotionProfileGenerator/3(v0 [m/s])  "<v0>"
  RampMotionProfileGenerator/2(VelocityRef [m/s]) -> MotionRefSelector/4(vCylRefGen [m])  "vCylRef [m]"
  Bus Selector/7 -> RampMotionProfileGenerator/8(tHoldPos [s])  "<tHoldPos>"
  Bus Selector/3 -> RampMotionProfileGenerator/4(Position_SP [m])  "<PosSP>"
  Bus Selector/4 -> RampMotionProfileGenerator/5("Velocity_SP [m/s] ")  "<VelSP>"
  MotionRefSelector/2(xCylRef [m]) -> DiscreteMotionControlSystem/5(PosRef [m]), Bus Creator1/3  "xCylRef [m]"
  Bus Selector/6 -> RampMotionProfileGenerator/7(tRamp [s])  "<tRamp>"
  Bool4/1 -> DiscreteMotionControlSystem/1(EnableVFF)  "EnableVFF"
  Bool6/1 -> DiscreteMotionControlSystem/2(Enable PFC)  "EnablePFC"
  Bool5/1 -> DiscreteMotionControlSystem/3(EnablePf)  "EnablePF"
  Bool7/1 -> RampMotionProfileGenerator/1(Enable), Switch1/2  "EnableMotion"
  Bus Selector/8 -> Time/1(<StartAuto>)  "<StartAuto>"
  Bus Selector/9 -> Time/2(<StopAuto>)  "<StopAuto>"

== system GreenCraneSimulator/Green Crane | Multibody System /Setup ==
  Mechanism Configuration1 : sm_lib/Utilities/Mechanism Configuration  UniformGravity=Constant  GravityVector=[0 0 -9.80665]  GravityUnits=m/s^2  LinearizationDelta=0.001  JointModeTransitionNonlinearIterations=2
  Solver Configuration : nesl_utility/Solver Configuration  PhysicalDomain=network_engine_domain  SubClassName=solver  LeftPortType=input  RightPortType=generic  Tones=[]  Harmonics=[]  SimulateNoise=off  Profile=off  UseLocalSampling=off  EnableSwitchedLinearOptims=on  FrequencyDomain=off  UseCCode=off  RelTol=0.001  AbsTol=1e-06  MinStep=1e-09  ToWorkspace=off  RevertToSquareIcSolve=off  NumHomotopyIterations=100  PhasorMode=off  PhasorModeNumHarmonics=1  DoDC=off  ResidualTolerance=1e-09  UseLocalSolver=off  LocalSolverChoice=NE_BACKWARD_EULER_ADVANCER  LocalSolverSampleTime=0.001  DoFixedCost=off  MaxNonlinIter=3  MaxModeIter=2  ComputeImpulses=off  ImpulseIterations=2  LinearAlgebra=Sparse  EquationFormulation=NE_TIME_EF  DelaysMemoryBudget=1024  AutomaticFiltering=on  FilteringTimeConstant=0.001  PartitionStorageMethod=AS_NEEDED  PartitionMemoryBudget=1024  PartitionMethod=FAST
      settings: SourceProductBaseCode=PW,SS
  World Frame : sm_lib/Frames and Transforms/World Frame
  Origin : PMIOPort  Side=Right
  connections:
  Solver Configuration/RConn1 -- World Frame/RConn1 -- Mechanism Configuration1/RConn1 -- Origin/RConn1

== system GreenCraneSimulator/Hydro-Mechanical System /Directional Control Valve ==
  u_dcv_ref [-] : Inport
  p_C [bar] : Inport  Port=2
  p_R [bar] : Inport  Port=3
  Edge Flows : Subsystem
  Edge Openings : Subsystem
  Gain : Gain  Gain=-1
  Load-Sensing Pressure : Subsystem
  Subtract3 : Sum  Inputs=-+
  Subtract4 : Sum  Inputs=+-
  Valve Dynamics : Subsystem
  Q_A1 [l/min] : Outport  VectorParamsAs1DForOutWhenUnconnected=off
  Q_B [l/min] : Outport  Port=2  VectorParamsAs1DForOutWhenUnconnected=off
  xDCV [-] : Outport  Port=3  VectorParamsAs1DForOutWhenUnconnected=off
  tag scope: p_LS=global
  wires:
  Valve Dynamics/1(u_dcv [-]) -> xDCV [-]/1, Load-Sensing Pressure/3(uDCV), Edge Openings/1(u_dcv [-])
  Edge Flows/2(Q_P-A [l/min]) -> Subtract3/2
  p_R [bar]/1 -> Edge Flows/8(p_R [bar])
  [p_A1] -> Load-Sensing Pressure/2(pA1), Edge Flows/6(p_A1 [bar])
  Subtract3/1 -> Q_A1 [l/min]/1
  Subtract4/1 -> Q_B [l/min]/1
  [p_B] -> Load-Sensing Pressure/1(pB), Edge Flows/7(p_B [bar])
  p_C [bar]/1 -> Edge Flows/5(p_C [bar])
  Edge Flows/4(Q_B-T [l/min]) -> Subtract4/2
  Edge Openings/2(u_A-T [-]) -> Edge Flows/2(u_A-T [-])  "u_A-T [-]"
  Edge Openings/4(u_P-B [-]) -> Edge Flows/4(u_P-B [-])  "u_P-B [-]"
  Edge Openings/1(u_B-T [-]) -> Edge Flows/1(u_B-T [-])  "u_B-T [-]"
  Edge Openings/3(u_P-A [-]) -> Edge Flows/3(u_P-A [-])  "u_P-A [-]"
  Edge Flows/3(Q_P-B [l/min]) -> Subtract4/1
  Edge Flows/1(Q_A-T [l/min]) -> Subtract3/1
  Load-Sensing Pressure/1(pLS) -> [p_LS]
  Gain/1 -> Valve Dynamics/1(u_dcv_ref [-])
  u_dcv_ref [-]/1 -> Gain/1

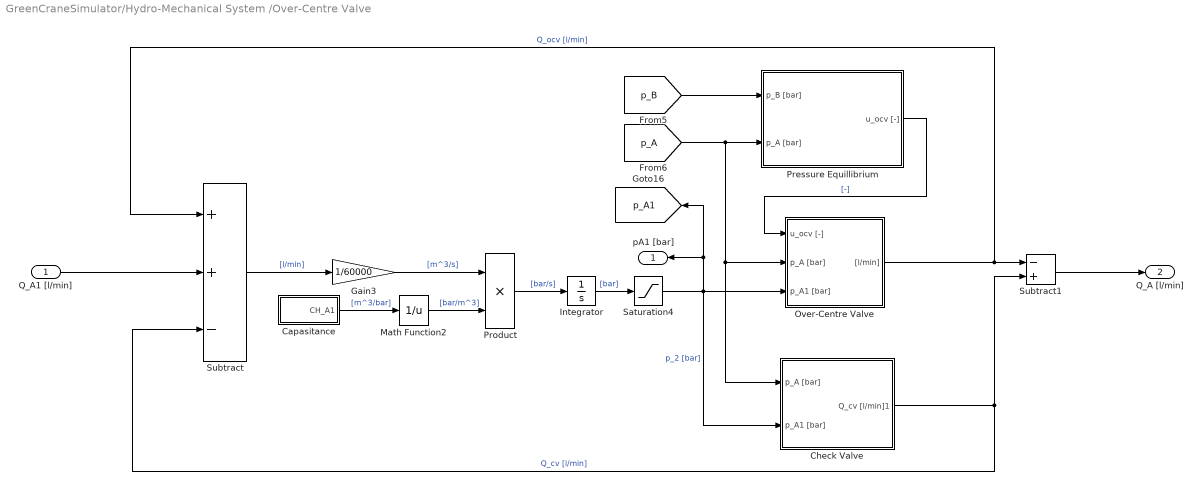
== system GreenCraneSimulator/Hydro-Mechanical System /Over-Centre Valve ==
  Q_A1 [l/min] : Inport
  Capasitance : Subsystem
  Check Valve : Subsystem
  Gain3 : Gain  Gain=1/60000
  Integrator : Integrator  InitialCondition=p0_A1
  Math Function2 : Math  Operator=reciprocal  SignedPower=on  SaturateOnIntegerOverflow=on
  Over-Centre Valve : Subsystem
  Pressure Equillibrium : Subsystem
  Product : Product
  Saturation4 : Saturate  UpperLimit=200  LowerLimit=p_R  ZeroCross=off
  Subtract : Sum  Inputs=++-
  Subtract1 : Sum  Inputs=-+
  pA1 [bar] : Outport  PortDimensions=1  VectorParamsAs1DForOutWhenUnconnected=off
  Q_A [l/min] : Outport  Port=2  PortDimensions=1  VectorParamsAs1DForOutWhenUnconnected=off
  tag scope: p_A1=global
  wires:
  [p_B] -> Pressure Equillibrium/1(p_B [bar])
  Pressure Equillibrium/1(u_ocv [-]) -> Over-Centre Valve/1(u_ocv [-])  "[-]"
  Check Valve/1(Q_cv [l/min]1) -> Subtract/3, Subtract1/2  "Q_cv [l/min]"
  Over-Centre Valve/1("[l/min]") -> Subtract1/1, Subtract/1  "Q_ocv [l/min]"
  Saturation4/1 -> Check Valve/2(p_A1 [bar]), Over-Centre Valve/3(p_A1 [bar]), pA1 [bar]/1, [p_A1]  "p_2 [bar]"
  Subtract/1 -> Gain3/1  "[l/min]"
  Q_A1 [l/min]/1 -> Subtract/2
  Product/1 -> Integrator/1  "[bar/s]"
  Integrator/1 -> Saturation4/1  "[bar]"
  Gain3/1 -> Product/1  "[m^3/s]"
  Subtract1/1 -> Q_A [l/min]/1
  [p_A] -> Pressure Equillibrium/2(p_A [bar]), Over-Centre Valve/2(p_A [bar]), Check Valve/1(p_A [bar])
  Capasitance/1("CH_A1 ") -> Math Function2/1  "[m^3/bar]"
  Math Function2/1 -> Product/2  "[bar/m^3]"

== system GreenCraneSimulator/Hydro-Mechanical System /Pressure Compensator1 ==
  p_S [bar] : Inport
  Compensator From Morten Bak Paper : MATLAB Function  TreatAsAtomicUnit=on
  "Compensator setting [bar] " : Constant  Value=p_pc_set
  Transfer Fcn1 : TransferFcn  Denominator=[tau_pc 1]
  p_C [bar] : Outport  VectorParamsAs1DForOutWhenUnconnected=off
  wires:
  [p_LS] -> Compensator From Morten Bak Paper/3(p_LS)
  "Compensator setting [bar] "/1 -> Compensator From Morten Bak Paper/1(p0)
  p_S [bar]/1 -> Compensator From Morten Bak Paper/2(p_S)
  Compensator From Morten Bak Paper/1(p_C) -> Transfer Fcn1/1  "p_C [bar]"
  Transfer Fcn1/1 -> p_C [bar]/1  "u_ocv_ref [-]"

== system GreenCraneSimulator/Hydro-Mechanical System /Rigid Mechanical System - Green Crane Arm ==
  note: Green Crane (Lagrangian mechanics)
  Force_Input : Inport
  Divide : Product  Inputs=*/
  Lasse Schmidt : MATLAB Function  TreatAsAtomicUnit=on
  Math Function : Math  Operator=square  SignedPower=on  SaturateOnIntegerOverflow=on
  Position : Integrator  InitialCondition=x_cyl_0
  Product : Product
  Scope : Scope
  Sum2 : Sum  Inputs=+--
  Velocity : Integrator  InitialCondition=v_cyl_0
  xCyl : Outport
  tag scope: v_cyl=global, x_cyl=global
  wires:
  Velocity/1 -> [v_cyl], Position/1, Math Function/1  "[m/s]"
  Lasse Schmidt/3(Meq) -> Divide/2  "[kg]"
  Sum2/1 -> Divide/1  "[N]"
  Force_Input/1 -> Sum2/1
  Divide/1 -> Velocity/1  "[m/s^2]"
  Lasse Schmidt/1(Geq) -> Sum2/2  "[N]"
  Position/1 -> xCyl/1, [x_cyl], Lasse Schmidt/1(x)  "[m]"
  Lasse Schmidt/2(Ceq) -> Product/1
  Math Function/1 -> Product/2
  Product/1 -> Sum2/3, Scope/1  "[N]"

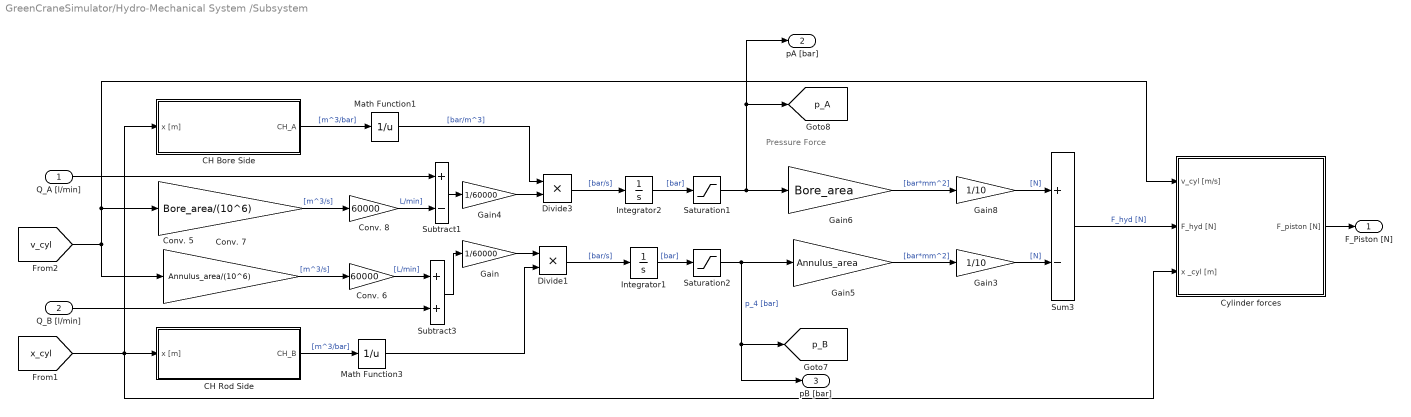
== system GreenCraneSimulator/Hydro-Mechanical System /Subsystem ==
  note: Pressure Force
  Q_A [l/min] : Inport
  Q_B [l/min] : Inport  Port=2
  CH Bore Side : Subsystem
  CH Rod Side : Subsystem
  Conv. 5 : Gain  Gain=Annulus_area/(10^6)
  Conv. 6 : Gain  Gain=60000
  Conv. 7 : Gain  Gain=Bore_area/(10^6)
  Conv. 8 : Gain  Gain=60000
  Cylinder forces : Subsystem
  Divide1 : Product  Inputs=**
  Divide3 : Product  Inputs=**
  Gain : Gain  Gain=1/60000
  Gain3 : Gain  Gain=1/10
  Gain4 : Gain  Gain=1/60000
  Gain5 : Gain  Gain=Annulus_area
  Gain6 : Gain  Gain=Bore_area
  Gain8 : Gain  Gain=1/10
  Integrator1 : Integrator  InitialCondition=p0_B  LowerSaturationLimit=0
  Integrator2 : Integrator  InitialCondition=p0_A  LowerSaturationLimit=0
  Math Function1 : Math  Operator=reciprocal  SignedPower=on  SaturateOnIntegerOverflow=on
  Math Function3 : Math  Operator=reciprocal  SignedPower=on  SaturateOnIntegerOverflow=on
  Saturation1 : Saturate  UpperLimit=200  LowerLimit=p_R  ZeroCross=off
  Saturation2 : Saturate  UpperLimit=200  LowerLimit=p_R  ZeroCross=off
  Subtract1 : Sum  Inputs=+-
  Subtract3 : Sum
  Sum3 : Sum  Inputs=+-
  F_Piston [N] : Outport  VectorParamsAs1DForOutWhenUnconnected=off
  pA [bar] : Outport  Port=2  VectorParamsAs1DForOutWhenUnconnected=off
  pB [bar] : Outport  Port=3  VectorParamsAs1DForOutWhenUnconnected=off
  tag scope: p_A=global, p_B=global
  wires:
  Sum3/1 -> Cylinder forces/2(F_hyd [N])  "F_hyd [N]"
  Gain8/1 -> Sum3/1  "[N]"
  Gain3/1 -> Sum3/2  "[N]"
  Saturation1/1 -> pA [bar]/1, [p_A], Gain6/1
  Gain5/1 -> Gain3/1  "[bar*mm^2]"
  Gain6/1 -> Gain8/1  "[bar*mm^2]"
  Cylinder forces/1(F_piston [N]) -> F_Piston [N]/1
  [v_cyl] -> Conv. 5/1, Cylinder forces/1(v_cyl [m/s]), Conv. 7/1
  [x_cyl] -> CH Rod Side/1(x [m]), CH Bore Side/1(x [m]), Cylinder forces/3(x _cyl [m])
  Integrator1/1 -> Saturation2/1  "[bar]"
  Q_B [l/min]/1 -> Subtract3/2
  Divide1/1 -> Integrator1/1  "[bar/s]"
  Saturation2/1 -> pB [bar]/1, [p_B], Gain5/1  "p_4 [bar]"
  Gain/1 -> Divide1/1
  Integrator2/1 -> Saturation1/1  "[bar]"
  Gain4/1 -> Divide3/2
  Divide3/1 -> Integrator2/1  "[bar/s]"
  Math Function1/1 -> Divide3/1  "[bar/m^3]"
  CH Bore Side/1(CH_A) -> Math Function1/1  "[m^3/bar]"
  Math Function3/1 -> Divide1/2
  CH Rod Side/1(CH_B) -> Math Function3/1  "[m^3/bar]"
  Subtract3/1 -> Gain/1
  Conv. 6/1 -> Subtract3/1  "[L/min]"
  Conv. 5/1 -> Conv. 6/1  "[m^3/s]"
  Subtract1/1 -> Gain4/1
  Q_A [l/min]/1 -> Subtract1/1
  Conv. 7/1 -> Conv. 8/1  "[m^3/s]"
  Conv. 8/1 -> Subtract1/2  "L/min]"

== system GreenCraneSimulator/PC | Ubuntu | ROS2/Green Crane | Visualizer  ==
  thetaBoom : Inport
  Boom : sm_lib/Body Elements/File Solid  ExtGeomFileName=..\Simulink Model MAS418 LAB #7\CAD\Boom.STL  UnitType=Custom  ExtGeomFileUnits=mm  StepReaderType=HEX  ExportConvexHullGeometry=off  InertiaType=CalculateFromGeometry  Mass=1  MassUnits=kg  CenterOfMass=[0 0 0]  CenterOfMassUnits=m  MomentsOfInertia=[1 1 1]  MomentsOfInertiaUnits=kg*m^2  ProductsOfInertia=[0 0 0]  ProductsOfInertiaUnits=kg*m^2  BasedOnType=Density  Density=1000  DensityUnits=kg/m^3  DoExposeReferenceFrame=off  SerializedFrames=<Frames><Frame><Id>Frame1</Id><Value><Name>F1</Name><Origin><Source>CenterOfMassFrame</Source><FeatureName></FeatureName></Origin><PrimaryAxis><DefinedDirection>+Y</DefinedDirection><Source>ReferenceFrame</Source><SourceDirection>-Z</SourceDirection><FeatureName></FeatureName></PrimaryAxis><SecondaryAxis><DefinedDirection>+X</DefinedDirection><Source>ReferenceFrame</Source><SourceDirection>+X</SourceDirection><FeatureName></FeatureName></SecondaryAxis></Value></Frame></Frames>  GraphicType=FromGeometry  MarkerShape=Sphere  MarkerSize=10  GraphicVisPropType=SimpleVisualProperties  GraphicDiffuseColor=[0.0 0.4 0.0]  GraphicSpecularColor=[0.5 0.5 0.5 1.0]  GraphicAmbientColor=[0.15 0.15 0.15 1.0]  GraphicEmissiveColor=[0.0 0.0 0.0 1.0]  GraphicShininess=75  GraphicOpacity=1.0
  Frame : sm_lib/Body Elements/File Solid  ExtGeomFileName=..\Simulink Model MAS418 LAB #7\CAD\Frame.STL  UnitType=Custom  ExtGeomFileUnits=mm  StepReaderType=HEX  ExportConvexHullGeometry=off  InertiaType=CalculateFromGeometry  Mass=1  MassUnits=kg  CenterOfMass=[0 0 0]  CenterOfMassUnits=m  MomentsOfInertia=[1 1 1]  MomentsOfInertiaUnits=kg*m^2  ProductsOfInertia=[0 0 0]  ProductsOfInertiaUnits=kg*m^2  BasedOnType=Density  Density=1000  DensityUnits=kg/m^3  DoExposeReferenceFrame=off  SerializedFrames=<Frames><Frame><Id>Frame1</Id><Value><Name>F1</Name><Origin><Source>CenterOfMassFrame</Source><FeatureName></FeatureName></Origin><PrimaryAxis><DefinedDirection>-Y</DefinedDirection><Source>ReferenceFrame</Source><SourceDirection>+Z</SourceDirection><FeatureName></FeatureName></PrimaryAxis><SecondaryAxis><DefinedDirection>+X</DefinedDirection><Source>ReferenceFrame</Source><SourceDirection>+X</SourceDirection><FeatureName></FeatureName></SecondaryAxis></Value></Frame></Frames>  GraphicType=FromGeometry  MarkerShape=Sphere  MarkerSize=10  GraphicVisPropType=SimpleVisualProperties  GraphicDiffuseColor=[0.0 0.4 0.0]  GraphicSpecularColor=[0.5 0.5 0.5 1.0]  GraphicAmbientColor=[0.15 0.15 0.15 1.0]  GraphicEmissiveColor=[0.0 0.0 0.0 1.0]  GraphicShininess=75  GraphicOpacity=1.0
  RJ Boom : sm_lib/Joints/Revolute Joint  JointMode=Normal  SenseConstraintForce=off  SenseConstraintForceX=off  SenseConstraintForceY=off  SenseConstraintForceZ=off  SenseConstraintTorque=off  SenseConstraintTorqueX=off  SenseConstraintTorqueY=off  SenseConstraintTorqueZ=off  SenseTotalForce=off  SenseTotalForceX=off  SenseTotalForceY=off  SenseTotalForceZ=off  SenseTotalTorque=off  SenseTotalTorqueX=off  SenseTotalTorqueY=off  SenseTotalTorqueZ=off  CompositeWrenchDir=FollowerOnBase  CompositeWrenchFrame=BaseFrame  EquilibriumPosition=0  EquilibriumPositionUnits=deg  SpringStiffness=0  SpringStiffnessUnits=N*m/deg  DampingCoefficient=0  DampingCoefficientUnits=N*m/(deg/s)  TorqueActuationMode=ComputedTorque  MotionActuationMode=InputMotion  SensePosition=off  SenseVelocity=off  SenseAcceleration=off  SenseTorqueForce=off  SenseLowerLimitTorqueForce=off  SenseUpperLimitTorqueForce=off  LowerLimitSpecify=off  LowerLimitBound=-90  LowerLimitBoundUnits=deg  LowerLimitStiffness=1e4  LowerLimitStiffnessUnits=N*m/deg  LowerLimitDamping=10  LowerLimitDampingUnits=N*m/(deg/s)  LowerLimitTransitionRegionWidth=0.1  LowerLimitTransitionRegionWidthUnits=deg  UpperLimitSpecify=off  UpperLimitBound=90  UpperLimitBoundUnits=deg  UpperLimitStiffness=1e4  UpperLimitStiffnessUnits=N*m/deg  UpperLimitDamping=10  UpperLimitDampingUnits=N*m/(deg/s)  UpperLimitTransitionRegionWidth=0.1  UpperLimitTransitionRegionWidthUnits=deg  PositionTargetSpecify=off  PositionTargetPriority=High  PositionTargetValue=0.326727675  PositionTargetValueUnits=rad  VelocityTargetSpecify=off  VelocityTargetPriority=High  VelocityTargetValue=0  VelocityTargetValueUnits=deg/s
  Rigid Transform : sm_lib/Frames and Transforms/Rigid Transform  TranslationMethod=Cartesian  TranslationStandardOffset=0  TranslationLengthUnit=mm  TranslationStandardAxis=+Z  TranslationCartesianOffset=[-568.76 0 1179.93]  TranslationROffset=0  TranslationROffsetUnits=m  TranslationZOffset=0  TranslationZOffsetUnits=m  TranslationThetaOffset=0  TranslationThetaOffsetUnits=deg  RotationMethod=StandardAxis  RotationAngleUnits=deg  RotationStandardAxis=+X  RotationAngle=90  RotationArbitraryAxis=[0 0 1]  FollAlignAxisA=+X  BaseAlignAxisA=+Y  FollAlignAxisB=+Y  BaseAlignAxisB=+Z  RotationSequenceAxes=FollowerAxes  RotationSequence=XYX  RotationSequenceAngles=[0 0 0]  RotationSequenceAnglesUnits=deg  RotationMatrix=[1 0 0; 0 1 0; 0 0 1]
  Rigid Transform1 : sm_lib/Frames and Transforms/Rigid Transform  TranslationMethod=Cartesian  TranslationStandardOffset=0  TranslationLengthUnit=mm  TranslationStandardAxis=+Z  TranslationCartesianOffset=[-3108.36 0 -63.43]  TranslationROffset=0  TranslationROffsetUnits=m  TranslationZOffset=0  TranslationZOffsetUnits=m  TranslationThetaOffset=0  TranslationThetaOffsetUnits=deg  RotationMethod=StandardAxis  RotationAngleUnits=deg  RotationStandardAxis=+X  RotationAngle=90  RotationArbitraryAxis=[0 0 1]  FollAlignAxisA=+X  BaseAlignAxisA=+Y  FollAlignAxisB=+Y  BaseAlignAxisB=+Z  RotationSequenceAxes=FollowerAxes  RotationSequence=XYX  RotationSequenceAngles=[0 0 0]  RotationSequenceAnglesUnits=deg  RotationMatrix=[1 0 0; 0 1 0; 0 0 1]
  Setup : Subsystem
  Simulink-PS Converter : nesl_utility/Simulink-PS Converter  PhysicalDomain=network_engine_domain  SubClassName=ps_input  LeftPortType=input  RightPortType=output  PseudoPeriodic=off  Frequencies=[]  NoiseDistribution=none  NoiseParameters=[]  Unit=1  AffineConversion=off  FilteringAndDerivatives=filter  SimscapeFilterOrder=2  InputFilterTimeConstant=0.001  UdotUserProvided=0
      settings: SourceProductBaseCode=PW,SS
  wires:
  thetaBoom/1 -> Simulink-PS Converter/1
  connections:
  Setup/RConn1 -- Rigid Transform/LConn1 -- Frame/LConn1
  Rigid Transform1/LConn1 -- Boom/LConn1
  RJ Boom/LConn1 -- Rigid Transform/RConn1
  RJ Boom/RConn1 -- Rigid Transform1/RConn1
  Simulink-PS Converter/RConn1 -- RJ Boom/LConn2

== system GreenCraneSimulator/PC | Ubuntu | ROS2/Scope ==
  In1 : Inport
  Demux : Demux  Outputs=13
  Flow : Scope
  Motion : Scope  NumInputPorts=3
  Mux : Mux  Inputs=2
  Mux1 : Mux  Inputs=2
  Mux2 : Mux  Inputs=3
  Mux3 : Mux  Inputs=2
  PLC Time : Display
  Pressures : Scope  NumInputPorts=2
  ValveOpening : Scope
  wires:
  Demux/4 -> Mux1/1  "xCyl [m]"
  Mux/1 -> Motion/1
  Demux/5 -> Mux/2  "vCylRef [m/s]"
  Demux/9 -> Mux2/2  "pr [bar]"
  Demux/3 -> Mux1/2  "xCylRef [m]"
  Mux1/1 -> Motion/2
  Demux/8 -> Mux2/1  "pp [bar]"
  Demux/7 -> ValveOpening/1  "xDCV [-]"
  Demux/2 -> Mux/1  "vCyl [m/s]"
  Demux/6 -> Motion/3  "xError [mm]"
  In1/1 -> Demux/1
  Demux/1 -> PLC Time/1
  Demux/10 -> Mux2/3  "pA [bar]"
  Mux2/1 -> Pressures/1
  Mux3/1 -> Pressures/2  "vCyl [m/s]"
  Demux/11 -> Mux3/1  "pS [bar]"
  Demux/12 -> Mux3/2  "pR [bar]"
  Demux/13 -> Flow/1  "Qr [l/min]"

== system GreenCraneSimulator/PLC/Discrete Derivative ==
  xCyl [m] : Inport
  Discrete Derivative : simulink/Discrete/Discrete Derivative  gainval=1.0  ICPrevScaledInput=0  OutMin=[]  OutMax=[]  OutDataType=fixdt(1, 16)  OutScaling=2^-10  DoSatur=off
  Saturation : Saturate
  Zero-Order Hold : ZeroOrderHold  SampleTime=tCycle
  vCyl [m/s] : Outport
  wires:
  Discrete Derivative/1 -> Saturation/1  "vCyl [m/s]"
  Zero-Order Hold/1 -> Discrete Derivative/1
  xCyl [m]/1 -> Zero-Order Hold/1
  Saturation/1 -> vCyl [m/s]/1  "vCyl [m/s]"
